simulink model "dc_motor_control"  (R2024a)
settings: Solver=VariableStepAuto  StartTime=0.0  StopTime=10.0  RelTol=1e-3
values from neighbouring files (symbols this model uses):
  A = [0 1 0 ... (first row only)    [main.m]
  A_sim = [0 1 0 ... (first row only)    [main.m]
  B = [0; 0; 1/L]    [main.m]
  B_sim = [0; 0; 1/L]    [main.m]
  C = [1 0 0]    [main.m]
  K_new = K_aug(1:3)    [main.m]
  Ki = -K_aug(4)    [main.m]
  Kt = 5.6627    [main.m]
  L = 0.0199    [main.m]
  N_int = K(1)/2    [main.m]
  R = 0.973    [main.m]
settings Model: Creator=Veli  LastModifiedBy=user
settings RTWCC: GPUComputeCapability=3.5

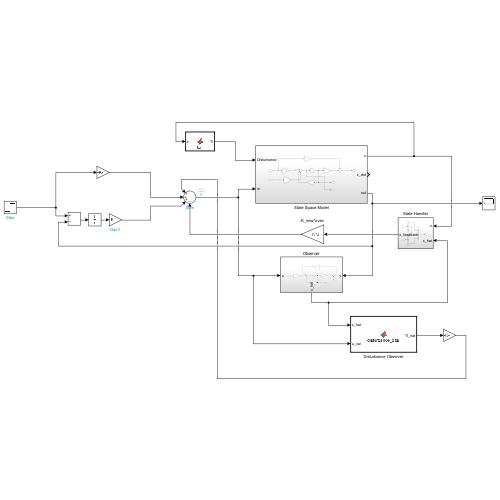
[thumbnail: Simulink's stored preview of the top-level diagram]
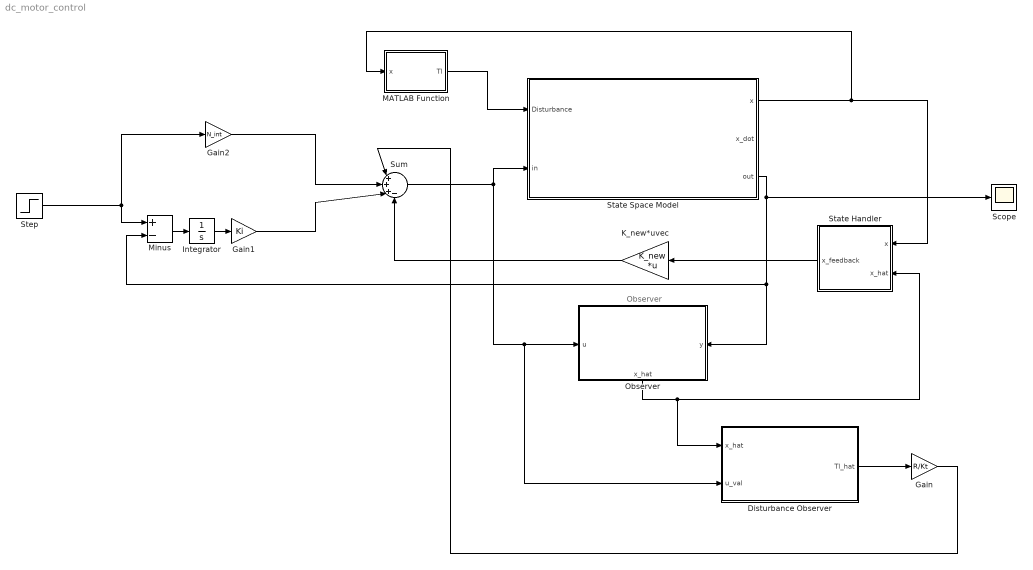
== system dc_motor_control ==
  note: Observer
  Disturbance Observer : MATLAB Function  TreatAsAtomicUnit=on
  Gain : Gain  Gain=R/Kt
  Gain1 : Gain  Gain=Ki
  Gain2 : Gain  Gain=N_int
  Integrator : Integrator
  K_new*uvec : Gain  Gain=K_new  Multiplication=Matrix(K*u)
  MATLAB Function : MATLAB Function  TreatAsAtomicUnit=on
  Minus : Sum  Inputs=+-
  Observer : Subsystem
      settings: PortSchema="{\"entries\":[{\"content\":{\"sides\":[{\"content\":{\"connectorIds\":[\"In1\"]},\"type\":\"ConnectorPlacement.EquallySpacedRectSide\",\"uuid\":\"173d3ed6-e0e9-4aa7-8bff-f85e206e3796\"},{\"content\":{\"connectorIds\":[\"In2\"],\"side\":\"RIGHT\"},\"type\":\"ConnectorPlacement.EquallySpacedRectSide\",\"uuid\":\"00ca6658-2383-49b1-9ba9-172b6a8f4637\"},{\"content\":{\"side\":\"TOP\"},\"type\":\"ConnectorPlacement.EquallySpacedRectSide\",\"uuid\":\"6401db1f-16eb-40b0-86f8-5f50cb70756a\"},{\"content\":{\"connectorIds\":[\"Out1\"],\"side\":\"BOTTOM\"},\"type\":\"ConnectorPlacement.EquallySpacedRectSide\",\"uuid\":\"72753f9d-ceb4-4321-8397-3b6f75796c34\"}]},\"type\":\"ConnectorPlacement.EquallySpacedConnector\",\"uuid\":\"b25a5a74-022c-41b1-aa34-c5d6fe8c6de1\"}],\"packageUris\":[\"http://schema.mathworks.com/mf0/Connector/R2020b\"],\"version\":\"1.0\"}"
  Scope : Scope
  State Handler : Subsystem
  State Space Model : Subsystem
  Step : Step  SampleTime=0
  Sum : Sum  Inputs=|+++-
  wires:
  K_new*uvec/1 -> Sum/4
  Sum/1 -> State Space Model/2(in), Disturbance Observer/2(u_val), Observer/1(u)
  State Space Model/3(out) -> Scope/1, Observer/2(y), Minus/2
  Step/1 -> Gain2/1, Minus/1
  State Space Model/1(x) -> MATLAB Function/1(x), State Handler/1(x)
  Observer/1(x_hat) -> Disturbance Observer/1(x_hat), State Handler/2(x_hat)
  State Handler/1(x_feedback) -> K_new*uvec/1
  Integrator/1 -> Gain1/1
  Minus/1 -> Integrator/1
  Gain1/1 -> Sum/3
  Gain2/1 -> Sum/2
  Disturbance Observer/1(Tl_hat) -> Gain/1
  Gain/1 -> Sum/1
  MATLAB Function/1(Tl) -> State Space Model/1(Disturbance)

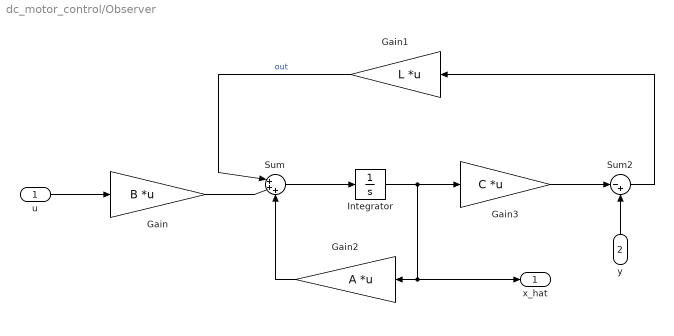
== system dc_motor_control/Observer ==
  u : Inport
  y : Inport  Port=2
  Gain : Gain  Gain=B  Multiplication=Matrix(K*u)
  Gain1 : Gain  Gain=L  Multiplication=Matrix(K*u)
  Gain2 : Gain  Gain=A  Multiplication=Matrix(K*u)
  Gain3 : Gain  Gain=C  Multiplication=Matrix(K*u)
  Integrator : Integrator
  Sum : Sum  Inputs=|+++
  Sum2 : Sum  Inputs=|-+
  x_hat : Outport
  wires:
  Gain3/1 -> Sum2/1
  Gain/1 -> Sum/2
  Gain2/1 -> Sum/3
  Sum/1 -> Integrator/1
  Integrator/1 -> Gain3/1, x_hat/1, Gain2/1
  y/1 -> Sum2/2
  Sum2/1 -> Gain1/1
  Gain1/1 -> Sum/1  "out"
  u/1 -> Gain/1

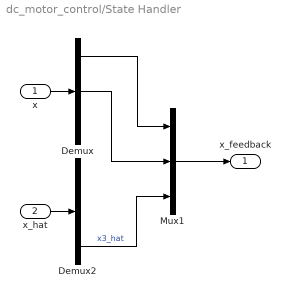
== system dc_motor_control/State Handler ==
  x : Inport
  x_hat : Inport  Port=2
  Demux : Demux  Outputs=3
  Demux2 : Demux  Outputs=3
  Mux1 : Mux  Inputs=3
  x_feedback : Outport
  wires:
  x/1 -> Demux/1
  Demux/1 -> Mux1/1
  x_hat/1 -> Demux2/1
  Demux/2 -> Mux1/2
  Demux2/3 -> Mux1/3  "x3_hat"
  Mux1/1 -> x_feedback/1

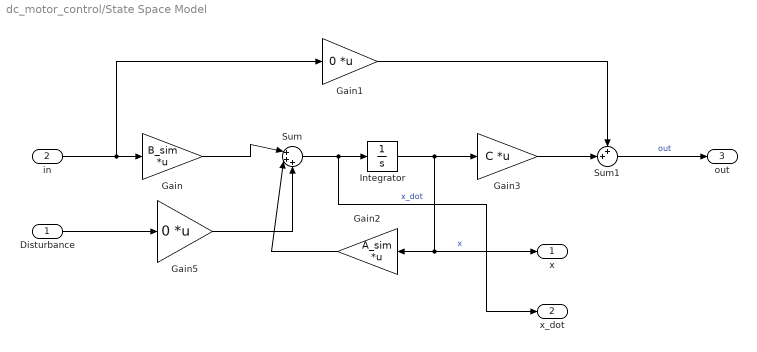
== system dc_motor_control/State Space Model ==
  Disturbance : Inport
  in : Inport  Port=2
  Gain : Gain  Gain=B_sim  Multiplication=Matrix(K*u)
  Gain1 : Gain  Gain=0  Multiplication=Matrix(K*u) (u vector)
  Gain2 : Gain  Gain=A_sim  Multiplication=Matrix(K*u)
  Gain3 : Gain  Gain=C  Multiplication=Matrix(K*u)
  Gain5 : Gain  Gain=0  Multiplication=Matrix(K*u)
  Integrator : Integrator
  Sum : Sum  Inputs=|+++
  Sum1 : Sum  Inputs=++|
  x : Outport
  x_dot : Outport  Port=2
  out : Outport  Port=3
  wires:
  Integrator/1 -> Gain3/1, x/1, Gain2/1  "x"
  Gain/1 -> Sum/1
  Disturbance/1 -> Gain5/1
  Sum/1 -> x_dot/1, Integrator/1  "x_dot"
  Gain3/1 -> Sum1/2
  Gain5/1 -> Sum/3
  Sum1/1 -> out/1  "out"
  Gain2/1 -> Sum/2
  Gain1/1 -> Sum1/1
  in/1 -> Gain1/1, Gain/1

== matlab function dc_motor_control/MATLAB Function ==
  data: x input; Tl output
function Tl = fcn(x)
    Tl = x(2) + 29.43 * sin(x(1));
end

== matlab function dc_motor_control/Disturbance Observer ==
  data: x_hat input; Tl_hat output; u_val input
function Tl_hat = disturbance_obs(x_hat, u_val)
    % Parametreler (Jeq=1.72 tasarım ataleti)
    bm = 4.6723;
    Kt = 5.6627;
    Jeq = 1.72;

    % x_hat(2) = hiz tahmini, x_hat(3) = akim tahmini
    % x2_dot tahminini durum uzayi denkleminden cekiyoruz:
    % x2_dot = (-bm/Jeq)*x2 + (Kt/Jeq)*x3
    x2_dot_hat = (-bm/Jeq)*x_hat(2) + (Kt/Jeq)*x_hat(3);

    % Yonergedeki Tl formulu 
    Tl_hat = 1.72 * x2_dot_hat + bm * x_hat(2) - Kt * x_hat(3);
end
